simulink model "db"  (R2018a)
settings: Solver=VariableStepAuto  StartTime=0.0  StopTime=1  MaxStep=1e-3  RelTol=1e-3
values from neighbouring files (symbols this model uses):
  A = 200    [codigo.m]
  fc = 0.136    [codigo.m]
  Jc = 0.136    [codigo.m]
  Jm = 1    [codigo.m]
  kb = 1    [codigo.m]
  ki = 1    [codigo.m]
  ks = 1    [codigo.m]
  La = 0.1    [codigo.m]
  n1 = 1    [codigo.m]
  n2 = 10    [codigo.m]
  Ra = 1    [codigo.m]
settings Model: Creator=carma  LastModifiedBy=carma

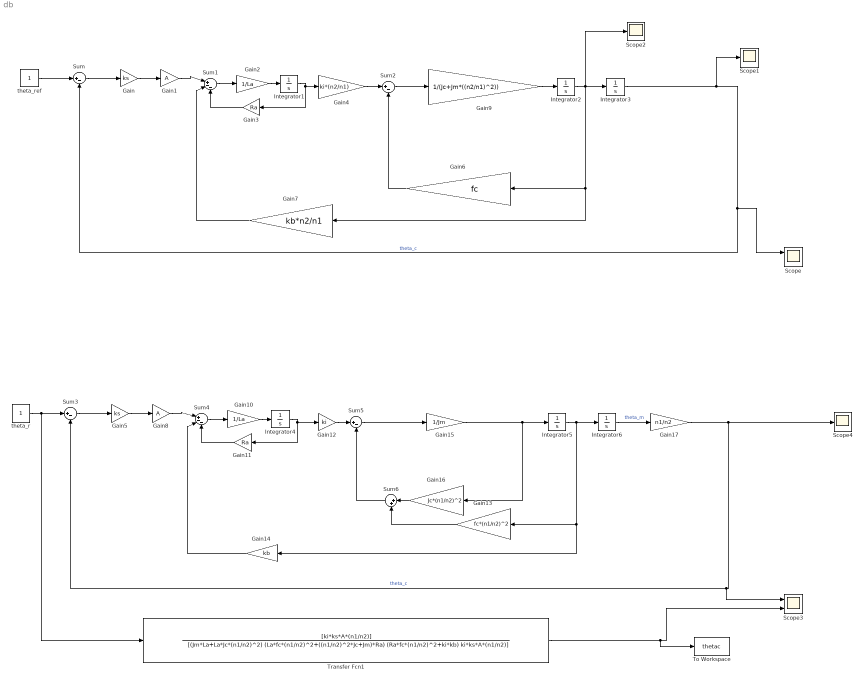
== system db ==
  Gain : Gain  Gain=ks
  Gain1 : Gain  Gain=A
  Gain10 : Gain  Gain=1/La
  Gain11 : Gain  Gain=Ra
  Gain12 : Gain  Gain=ki
  Gain13 : Gain  Gain=fc*(n1/n2)^2
  Gain14 : Gain  Gain=kb
  Gain15 : Gain  Gain=1/Jm
  Gain16 : Gain  Gain=Jc*(n1/n2)^2
  Gain17 : Gain  Gain=n1/n2
  Gain2 : Gain  Gain=1/La
  Gain3 : Gain  Gain=Ra
  Gain4 : Gain  Gain=ki*(n2/n1)
  Gain5 : Gain  Gain=ks
  Gain6 : Gain  Gain=fc
  Gain7 : Gain  Gain=kb*n2/n1
  Gain8 : Gain  Gain=A
  Gain9 : Gain  Gain=1/(Jc+Jm*((n2/n1)^2))
  Integrator{1..6} (6 alike) : Integrator
  Scope : Scope  NumInputPorts=2
  Scope1 : Scope
  Scope2 : Scope
  Scope3 : Scope  NumInputPorts=2
  Scope4 : Scope
  Sum{,2..3,5} (4 alike) : Sum  Inputs=|+-
  Sum1 : Sum  Inputs=|+--
  Sum4 : Sum  Inputs=|+--
  Sum6 : Sum  Inputs=|++
  To Workspace : ToWorkspace  VariableName=thetac  SampleTime=1e-3
  Transfer Fcn1 : TransferFcn  Numerator=[ki*ks*A*(n1/n2)]  Denominator=[(Jm*La+La*Jc*(n1/n2)^2) (La*fc*(n1/n2)^2+((n1/n2)^2*Jc+Jm)*Ra) (Ra*fc*(n1/n2)^2+ki*kb) ki*ks*A*(n1/n2)]
  theta_r : Constant
  theta_ref : Constant
  wires:
  theta_ref/1 -> Sum/1
  Integrator3/1 -> Scope1/1, Scope/1, Sum/2  "theta_c"
  Sum/1 -> Gain/1
  Gain/1 -> Gain1/1
  Gain2/1 -> Integrator1/1
  Gain1/1 -> Sum1/1
  Sum1/1 -> Gain2/1
  Integrator1/1 -> Gain3/1, Gain4/1
  Gain3/1 -> Sum1/3
  Gain4/1 -> Sum2/1
  Sum2/1 -> Gain9/1
  Integrator2/1 -> Scope2/1, Integrator3/1, Gain7/1, Gain6/1
  Gain7/1 -> Sum1/2
  Gain9/1 -> Integrator2/1
  Gain6/1 -> Sum2/2
  theta_r/1 -> Transfer Fcn1/1, Sum3/1
  Gain14/1 -> Sum4/2
  Gain8/1 -> Sum4/1
  Sum5/1 -> Gain15/1
  Gain15/1 -> Gain16/1, Integrator5/1
  Gain12/1 -> Sum5/1
  Integrator5/1 -> Integrator6/1, Gain14/1, Gain13/1
  Gain11/1 -> Sum4/3
  Gain10/1 -> Integrator4/1
  Sum3/1 -> Gain5/1
  Gain5/1 -> Gain8/1
  Integrator6/1 -> Gain17/1  "theta_m"
  Integrator4/1 -> Gain12/1, Gain11/1
  Sum4/1 -> Gain10/1
  Gain16/1 -> Sum6/1
  Sum6/1 -> Sum5/2
  Gain13/1 -> Sum6/2
  Gain17/1 -> Scope4/1, Scope3/1, Sum3/2  "theta_c"
  Transfer Fcn1/1 -> To Workspace/1, Scope3/2
